simulink model "Doppelpendel_LQR"  (R2020b)
settings: Solver=ode45  StartTime=0.0  StopTime=10.0  RelTol=1e-3
values from neighbouring files (symbols this model uses):
  parLQR = LQR_Entwurf(sysd,parLQR)    [loesung.m]
  Quantisierung = 1    [LoadParameter.m]
undefined symbols (not defined in the file or in its folder): parDP
libraries: cstblocks x3
settings Model: Creator=tg  LastModifiedBy=Armin Wessel
settings DataIOCC: LimitDataPoints=on  SaveFormat=Array  ReturnWorkspaceOutputs=off
settings OptimizationCC: BlockReduction=off  BooleanDataType=off  LifeSpan=inf
settings DebuggingCC: SaveWithParameterizedLinksMsg=none  UnderspecifiedInitializationDetection=Classic  MergeDetectMultiDrivingBlocksExec=none  SignalResolutionControl=TryResolveAllWithWarning  AllowSymbolicDim=off  SFUnexpectedBacktrackingDiag=warning  SFNoUnconditionalDefaultTransitionDiag=warning  SFExecutionAtInitializationDiag=none  ArithmeticOperatorsInVariantConditions=warning
settings HardwareCC: ProdBitPerPointer=32  ProdBitPerSizeT=32  ProdBitPerPtrDiffT=32  ProdLargestAtomicFloat=None  ProdIntDivRoundTo=Undefined  ProdEndianess=Unspecified  ProdWordSize=32  ProdHWDeviceType=32-bit Generic  TargetUnknown=on
settings ModelReferenceCC: PropagateSignalLabelsOutOfModel=off
settings SFSimCC: SimUseLocalCustomCode=off  CustomCodeUndefinedFunction=UseInterfaceOnly
settings RTWCC: RTWUseLocalCustomCode=off
settings CodeAppCC: StateflowObjectComments=on
settings GRTTargetCC: TargetLangStandard=C89/C90 (ANSI)
settings ConfigComp: CovMetricSettings=dw  CovSaveCumulativeToWorkspaceVar=on  CovSaveSingleToWorkspaceVar=on  CovExternalEMLEnable=off

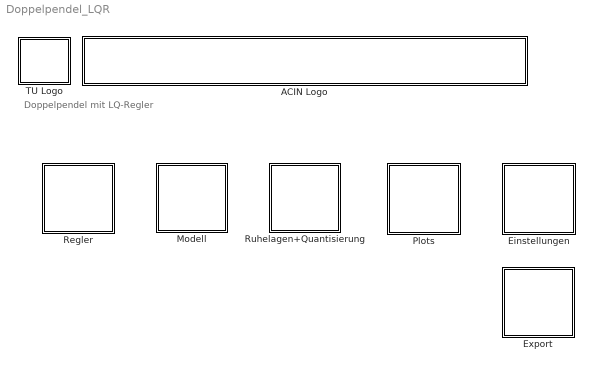
== system Doppelpendel_LQR ==
  note: Doppelpendel mit LQ-Regler
  ACIN Logo : Subsystem
      mask init:
      | s = get_param(gcb,'UserData');
      mask Display:
      | image(s.logo,[0 0 439 45]);
      | %axis image
  Einstellungen : Subsystem
  Export : Subsystem
  Modell : Subsystem
  Plots : Subsystem
  Regler : Subsystem
  Ruhelagen+Quantisierung : Subsystem
  TU Logo : Subsystem
      mask init:
      | s = get_param(gcb,'UserData');
      mask Display: image(s.logo,[0 0 45 45]);

== system Doppelpendel_LQR/ACIN Logo ==

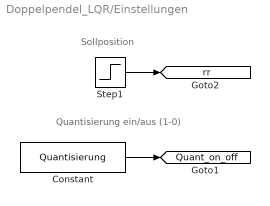
== system Doppelpendel_LQR/Einstellungen ==
  note: Sollposition
  note: Quantisierung ein/aus (1-0)
  Constant : Constant  Value=Quantisierung
  Step1 : Step  Time=3  After=0.1  SampleTime=parLQR.Ta
  tag scope: Quant_on_off=global, rr=global
  wires:
  Step1/1 -> [rr]
  Constant/1 -> [Quant_on_off]

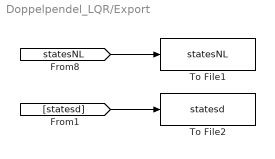
== system Doppelpendel_LQR/Export ==
  To File1 : ToFile  Filename=statesNL  MatrixName=data  SampleTime=parDP.Ta
  To File2 : ToFile  Filename=statesd  MatrixName=data  SampleTime=parDP.Ta
  wires:
  [statesNL] -> To File1/1
  [statesd] -> To File2/1

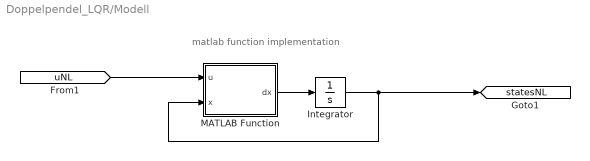
== system Doppelpendel_LQR/Modell ==
  note: matlab function implementation
  Integrator : Integrator  InitialCondition=parDP.IC
  MATLAB Function : MATLAB Function  TreatAsAtomicUnit=on
  tag scope: statesNL=global
  wires:
  Integrator/1 -> [statesNL], MATLAB Function/2(x)
  [uNL] -> MATLAB Function/1(u)
  MATLAB Function/1(dx) -> Integrator/1

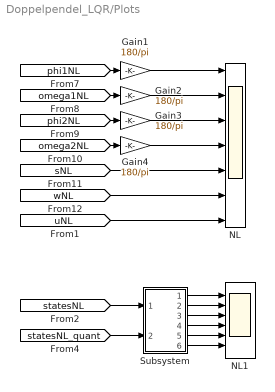
== system Doppelpendel_LQR/Plots ==
  Gain{1..4} (4 alike) : Gain  Gain=180/pi
  NL : Scope  NumInputPorts=7
  NL1 : Scope  NumInputPorts=6
  Subsystem : Subsystem
  wires:
  [omega1NL] -> Gain2/1
  [omega2NL] -> Gain4/1
  [sNL] -> NL/5
  [wNL] -> NL/6
  Gain1/1 -> NL/1
  Gain2/1 -> NL/2
  Gain3/1 -> NL/3
  Gain4/1 -> NL/4
  [phi1NL] -> Gain1/1
  [phi2NL] -> Gain3/1
  [statesNL] -> Subsystem/1(In1)
  [statesNL_quant] -> Subsystem/2(In2)
  Subsystem/1(Out1) -> NL1/1
  Subsystem/2(Out2) -> NL1/2
  Subsystem/3(Out3) -> NL1/3
  Subsystem/4(Out4) -> NL1/4
  Subsystem/5(Out5) -> NL1/5
  Subsystem/6(Out6) -> NL1/6
  [uNL] -> NL/7

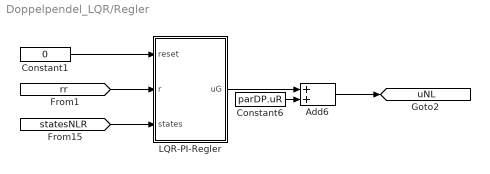
== system Doppelpendel_LQR/Regler ==
  Add6 : Sum
  Constant1 : Constant  Value=0
  Constant6 : Constant  Value=parDP.uR
  LQR-PI-Regler : MATLAB Function  TreatAsAtomicUnit=on
  tag scope: uNL=global
  wires:
  Constant6/1 -> Add6/2
  Add6/1 -> [uNL]
  LQR-PI-Regler/1(uG) -> Add6/1
  [statesNLR] -> LQR-PI-Regler/3(states)
  [rr] -> LQR-PI-Regler/2(r)
  Constant1/1 -> LQR-PI-Regler/1(reset)

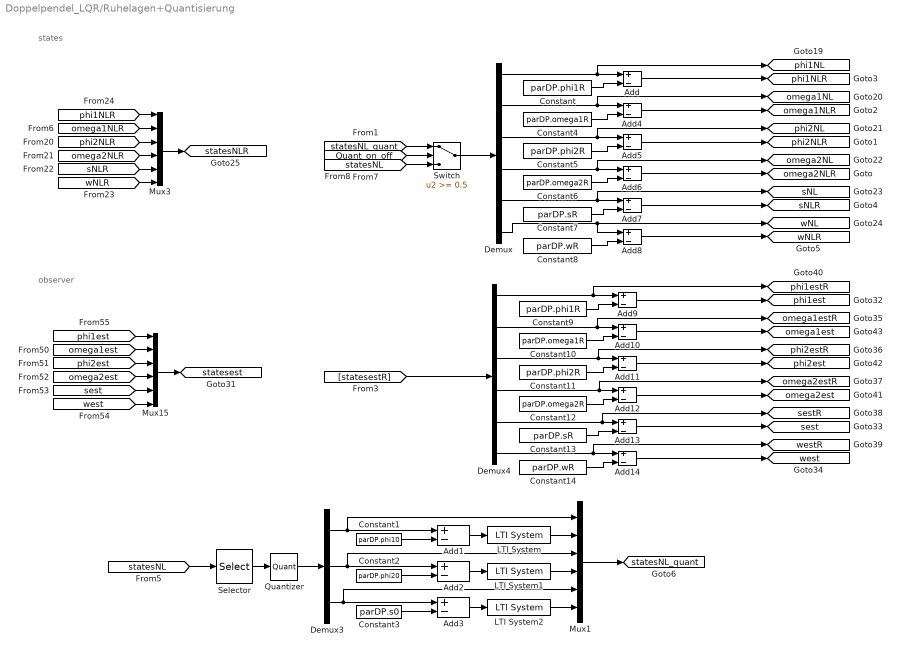
== system Doppelpendel_LQR/Ruhelagen+Quantisierung ==
  note: observer
  note: states
  Add{,1..14} (15 alike) : Sum  Inputs=+-
  Constant : Constant  Value=parDP.phi1R
  Constant1 : Constant  Value=parDP.phi10
  Constant10 : Constant  Value=parDP.omega1R
  Constant11 : Constant  Value=parDP.phi2R
  Constant12 : Constant  Value=parDP.omega2R
  Constant13 : Constant  Value=parDP.sR
  Constant14 : Constant  Value=parDP.wR
  Constant2 : Constant  Value=parDP.phi20
  Constant3 : Constant  Value=parDP.s0
  Constant4 : Constant  Value=parDP.omega1R
  Constant5 : Constant  Value=parDP.phi2R
  Constant6 : Constant  Value=parDP.omega2R
  Constant7 : Constant  Value=parDP.sR
  Constant8 : Constant  Value=parDP.wR
  Constant9 : Constant  Value=parDP.phi1R
  Demux : Demux  Outputs=6
  Demux3 : Demux  Outputs=3
  Demux4 : Demux  Outputs=6
  LTI System : cstblocks/LTI System  sys=Fd_diff  IC=[]
  LTI System1 : cstblocks/LTI System  sys=Fd_diff  IC=[]
  LTI System2 : cstblocks/LTI System  sys=Fd_diff  IC=[]
  Mux1 : Mux  Inputs=6
  Mux15 : Mux  Inputs=6
  Mux3 : Mux  Inputs=6
  Quantizer : Quantizer  QuantizationInterval=Phiquantisierung  SampleTime=parLQR.Ta
  Selector : Selector  InputPortWidth=6  IndexOptions=Index vector (dialog)  Indices=[1 3 5]  OutputSizes=1
  Switch : Switch  Threshold=0.5
  tag scope: omega1NL=global, omega1NLR=global, omega1est=global, omega1estR=global, omega2NL=global, omega2NLR=global, omega2est=global, omega2estR=global, phi1NL=global, phi1NLR=global, phi1est=global, phi1estR=global, phi2NL=global, phi2NLR=global, phi2est=global, phi2estR=global, sNL=global, sNLR=global, sest=global, sestR=global, statesNLR=global, statesNL_quant=global, statesest=global, wNL=global, wNLR=global, west=global, westR=global
  wires:
  [phi1NLR] -> Mux3/1
  [omega1NLR] -> Mux3/2
  [phi2NLR] -> Mux3/3
  [omega2NLR] -> Mux3/4
  [sNLR] -> Mux3/5
  [wNLR] -> Mux3/6
  Mux3/1 -> [statesNLR]
  [phi1est] -> Mux15/1
  [omega1est] -> Mux15/2
  [phi2est] -> Mux15/3
  [omega2est] -> Mux15/4
  [sest] -> Mux15/5
  [west] -> Mux15/6
  Mux15/1 -> [statesest]
  [statesNL] -> Selector/1
  Mux1/1 -> [statesNL_quant]
  LTI System/1 -> Mux1/2
  LTI System2/1 -> Mux1/6
  LTI System1/1 -> Mux1/4
  Add1/1 -> LTI System/1
  Add2/1 -> LTI System1/1
  Add3/1 -> LTI System2/1
  Constant1/1 -> Add1/2
  Constant2/1 -> Add2/2
  Constant3/1 -> Add3/2
  Demux3/3 -> Add3/1, Mux1/5
  Demux3/2 -> Add2/1, Mux1/3
  Demux3/1 -> Add1/1, Mux1/1
  [statesestR] -> Demux4/1
  Switch/1 -> Demux/1
  [statesNL] -> Switch/3
  [Quant_on_off] -> Switch/2
  [statesNL_quant] -> Switch/1
  Quantizer/1 -> Demux3/1
  Selector/1 -> Quantizer/1
  Add8/1 -> [wNLR]
  Constant8/1 -> Add8/2
  Constant6/1 -> Add6/2
  Add4/1 -> [omega1NLR]
  Demux/6 -> Add8/1, [wNL]
  Constant7/1 -> Add7/2
  Add7/1 -> [sNLR]
  Add6/1 -> [omega2NLR]
  Demux/1 -> [phi1NL], Add/1
  Demux/4 -> [omega2NL], Add6/1
  Constant4/1 -> Add4/2
  Add5/1 -> [phi2NLR]
  Constant5/1 -> Add5/2
  Demux/2 -> [omega1NL], Add4/1
  Demux/3 -> [phi2NL], Add5/1
  Add/1 -> [phi1NLR]
  Demux/5 -> [sNL], Add7/1
  Constant/1 -> Add/2
  Demux4/1 -> [phi1estR], Add9/1
  Constant10/1 -> Add10/2
  Demux4/2 -> [omega1estR], Add10/1
  Add11/1 -> [phi2est]
  Add13/1 -> [sest]
  Constant13/1 -> Add13/2
  Constant11/1 -> Add11/2
  Add14/1 -> [west]
  Constant12/1 -> Add12/2
  Demux4/6 -> [westR], Add14/1
  Demux4/4 -> Add12/1, [omega2estR]
  Add10/1 -> [omega1est]
  Constant14/1 -> Add14/2
  Add9/1 -> [phi1est]
  Demux4/3 -> Add11/1, [phi2estR]
  Add12/1 -> [omega2est]
  Constant9/1 -> Add9/2
  Demux4/5 -> Add13/1, [sestR]

== system Doppelpendel_LQR/TU Logo ==

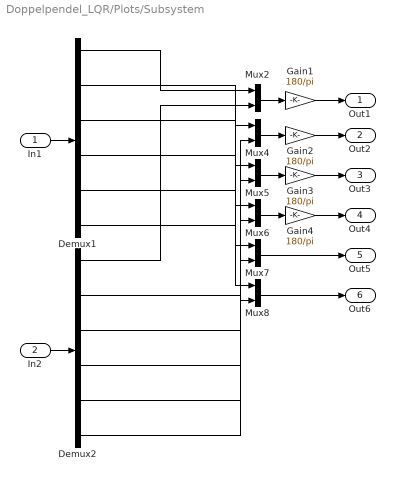
== system Doppelpendel_LQR/Plots/Subsystem ==
  In1 : Inport
  In2 : Inport  Port=2
  Demux1 : Demux  Outputs=6
  Demux2 : Demux  Outputs=6
  Gain{1..4} (4 alike) : Gain  Gain=180/pi
  Mux{2,4..8} (6 alike) : Mux  Inputs=2
  Out1 : Outport  VectorParamsAs1DForOutWhenUnconnected=off
  Out2 : Outport  Port=2  VectorParamsAs1DForOutWhenUnconnected=off
  Out3 : Outport  Port=3  VectorParamsAs1DForOutWhenUnconnected=off
  Out4 : Outport  Port=4  VectorParamsAs1DForOutWhenUnconnected=off
  Out5 : Outport  Port=5  VectorParamsAs1DForOutWhenUnconnected=off
  Out6 : Outport  Port=6  VectorParamsAs1DForOutWhenUnconnected=off
  wires:
  Demux1/1 -> Mux2/1
  Demux2/1 -> Mux2/2
  Demux2/2 -> Mux4/2
  Demux2/3 -> Mux5/2
  Demux2/4 -> Mux6/2
  Demux2/5 -> Mux7/2
  Demux2/6 -> Mux8/2
  Demux1/6 -> Mux8/1
  Demux1/5 -> Mux7/1
  Demux1/2 -> Mux4/1
  Demux1/3 -> Mux5/1
  Demux1/4 -> Mux6/1
  Mux2/1 -> Gain1/1
  Mux4/1 -> Gain2/1
  In1/1 -> Demux1/1
  Mux5/1 -> Gain3/1
  Mux6/1 -> Gain4/1
  Mux7/1 -> Out5/1
  Mux8/1 -> Out6/1
  In2/1 -> Demux2/1
  Gain1/1 -> Out1/1
  Gain2/1 -> Out2/1
  Gain3/1 -> Out3/1
  Gain4/1 -> Out4/1

== matlab function Doppelpendel_LQR/Modell/MATLAB Function ==
  data: u input; dx output; x input; parDP parameter
function dx = fcnDoppelpendel(u,x,parDP)
    %#codegen
    % calculates rhs of ODE
    dx = Doppelpendel_NL_mfun(u,x,parDP);
end

== matlab function Doppelpendel_LQR/Regler/LQR-PI-Regler ==
  settings: updateMethod=DISCRETE  sampleTime=parLQR.Ta
  data: reset input; r input; states input; uG output; parLQR parameter
function uG  = LQR(reset,r,states,parLQR)
%Anfangsbedingung I-Anteil
persistent xI

if isempty(xI) xI = double(0); end
% Folgendes hier bitte ausführen:
% 1.) PI-Zustandsregler einfügen
% 2.) if (reset==1) xI=0; end

xI = xI+(r-states(5));

if (reset==1) 
    xI=0; 
end

%Gesamtrückführung
uG=[parLQR.kx, parLQR.kI]*[states; xI];
